simulink model "tester"  (R2020a)
settings: Solver=VariableStepAuto  StartTime=0.0  StopTime=inf  RelTol=1e-3
libraries: robotlib x2
settings Model: Creator=root  LastModifiedBy=root

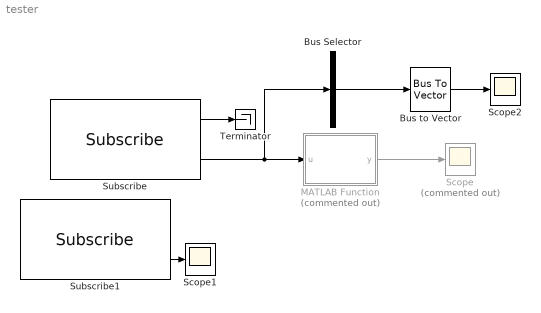
== system tester ==
  Bus Selector : BusSelector  OutputSignals=Groundtruth  OutputAsBus=on
  Bus to Vector : BusToVector
  MATLAB Function : MATLAB Function  Commented=on  TreatAsAtomicUnit=on
  Scope : Scope  Commented=on
  Scope1 : Scope
  Scope2 : Scope
  Subscribe : robotlib/Subscribe  topicSource=Select from ROS network  topic=/radar_processed_array  messageType=radar_msgs/RadarProcessedArray  sampleTime=-1  messageQueueLength=1
  Subscribe1 : robotlib/Subscribe  topicSource=Select from ROS network  topic=/clock  messageType=rosgraph_msgs/Clock  sampleTime=-1  messageQueueLength=1
  Terminator : Terminator
  wires:
  Subscribe/1 -> Terminator/1
  Subscribe/2 -> Bus Selector/1, MATLAB Function/1(u)
  MATLAB Function/1(y) -> Scope/1
  Subscribe1/2 -> Scope1/1
  Bus Selector/1 -> Bus to Vector/1
  Bus to Vector/1 -> Scope2/1

== matlab function tester/MATLAB Function ==
  data: u input; y output
function y = Range(u)

i = 1;
y = -10;

while (i < length(u.Groundtruth))
    %fprintf("%f, %f\n",radar_proc_data.Groundtruth(i,1).ObjectType, radar_proc_data.Groundtruth(i,1).Range)
    range = u.Groundtruth(i,1).Range;
    object_type = u.Groundtruth(i,1).ObjectType;
    if (object_type == 2.0)
        y = range;
    end
    i = 1 + 1;
end

end
